simulink model "logic_gate"  (R2021b)
settings: Solver=VariableStepAuto  StartTime=0.0  StopTime=10.0  RelTol=1e-3
settings Model: Creator=soper  LastModifiedBy=soper

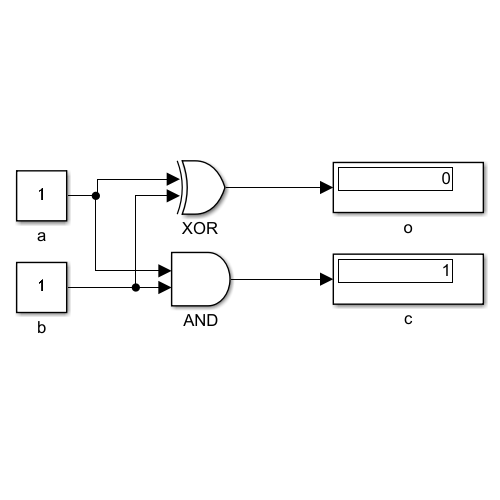
[thumbnail: Simulink's stored preview of the top-level diagram]
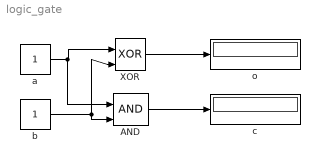
== system logic_gate ==
  AND : Logic  IconShape=distinctive  AllPortsSameDT=off  OutDataTypeStr=boolean
  XOR : Logic  Operator=XOR  IconShape=distinctive  AllPortsSameDT=off  OutDataTypeStr=boolean
  a : Constant
  b : Constant
  c : Display
  o : Display
  wires:
  b/1 -> AND/2, XOR/2
  AND/1 -> c/1
  XOR/1 -> o/1
  a/1 -> AND/1, XOR/1
